simulink model "simulation"  (R2024b)
settings: Solver=FixedStepDiscrete  StartTime=0.0  StopTime=4  FixedStep=Ts  MaxStep=0.0001  RelTol=1e-3
PreLoadFcn:
  | load('parameters.m')
  | load('motor_parameters.m')
InitFcn:
  | if ~ evalin('base', 'exist(''A2'', ''var'')')
  |     load('all_parameters.mat');
  | end
values from neighbouring files (symbols this model uses):
  A1a = [0  0.0011361488425; -0.0011361488425  0]    [all_parameters.mat]    (also in parameters.m = [0 a12; a21 0])
  A1d = [0.987343830616  0; 0  0.987343830616]    [all_parameters.mat]    (also in parameters.m = [a11 0; 0 a22])
  A2 = [0.87358490566  0; 0  0.87358490566]    [all_parameters.mat]    (also in parameters.m = [a33, 0; 0, a44])
  A3a = [0  -0.00121090521585; 0.00121090521585  0]    [all_parameters.mat]    (also in parameters.m = [0 a52; a61 0])
  A3d = [-0.0123977153824  0; 0  -0.0123977153824]    [all_parameters.mat]    (also in parameters.m = [a51 0; 0 a62])
  B1 = [0.00755592202018  0; 0  0.00755592202018]    [all_parameters.mat]    (also in parameters.m = [b1, 0; 0, b1]*4)
  B1_inv = [132.346522017  0; 0  132.346522017]    [all_parameters.mat]    (also in parameters.m = inv(B1))
  B2 = [0.0188679245283  0; 0  0.0188679245283]    [all_parameters.mat]    (also in parameters.m = [b2, 0; 0, b2])
  B2_inv = [53  0; 0  53]    [all_parameters.mat]    (also in parameters.m = inv(B2))
  B3 = [-0.00740162112379  0; 0  -0.00740162112379]    [all_parameters.mat]    (also in parameters.m = [b3, 0; 0, b3]*4)
  Bm = 0.0024    [all_parameters.mat]    (also in parameters.m)
  gamma = [0.9  0; 0  0.9]    [all_parameters.mat]    (also in parameters.m = diag(v_gamma))
  H1a = [0  0.0011598340301; -0.0011598340301  0]    [all_parameters.mat]    (also in parameters.m = [0 h12; h21 0])
  H1d = [0.0127677964385  0; 0  0.0127677964385]    [all_parameters.mat]    (also in parameters.m = [h11 0; 0 h22])
  H2a = [0  -0.0012361488425; 0.0012361488425  0]    [all_parameters.mat]    (also in parameters.m = [0 h32; h41 0])
  H2d = [0.986392107509  0; 0  0.986392107509]    [all_parameters.mat]    (also in parameters.m = [h31 0; 0 h42])
  Jm_ = 2.38095238095    [all_parameters.mat]    (also in parameters.m)
  lambda = [0.5  0; 0  0.5]    [all_parameters.mat]    (also in parameters.m = diag(v_lambda))
  Lr = 0.6268    [all_parameters.mat]    (also in parameters.m)
  M_ind = 0.1535    [all_parameters.mat]    (also in parameters.m)
  P = 1    [all_parameters.mat]    (also in parameters.m)
  rho = [30  0; 0  30]    [all_parameters.mat]    (also in parameters.m = [rho1 0; 0 rho2])
  Rr = 6.9    [all_parameters.mat]    (also in parameters.m)
  T_inv = [1 0.866025403784 -0.5 -0.866025403784 -0.5 0 0 0.5 0.866025403784 0.5 -0.866025403784 -1 ... (36 elements, 6x6)]    [all_parameters.mat]    (also in parameters.m = inv(T))
  Tl = 2    [all_parameters.mat]    (also in parameters.m)
  Ts = 0.0001    [all_parameters.mat]    (also in parameters.m)
undefined symbols (not defined in the file or in its folder): rad, s
libraries: aerolibconvert2 x2, simulink x2, slpidlib x1, mcbcontrolslib x1
settings Model: Creator=bojack  LastModifiedBy=bojack

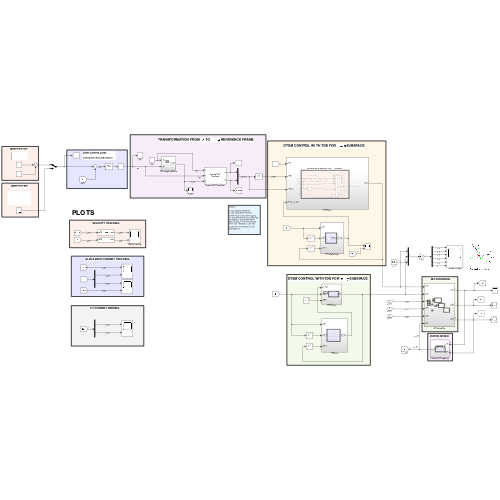
[thumbnail: Simulink's stored preview of the top-level diagram]
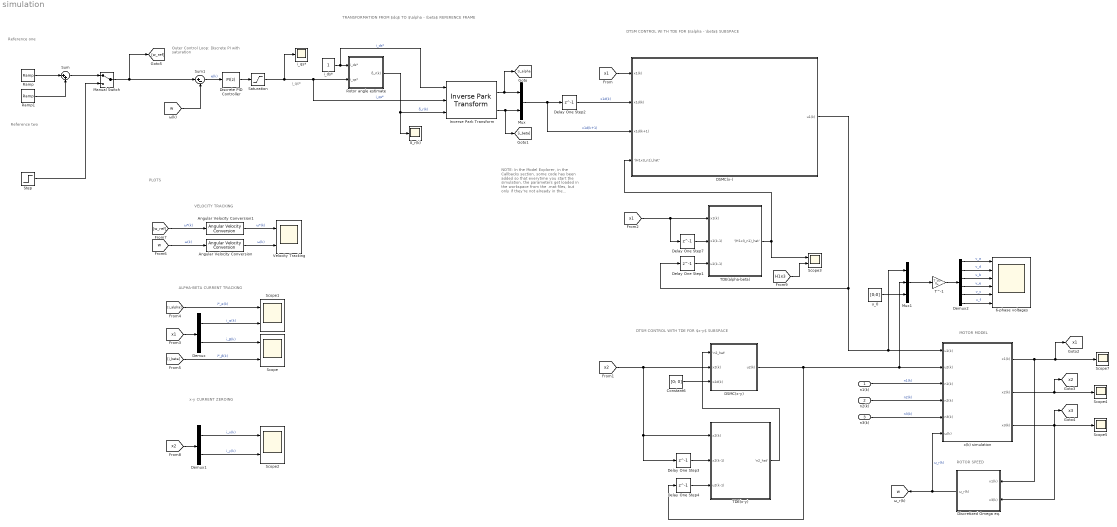
== system simulation ==
  note: Reference one
  note: VELOCITY TRACKING
  note: PLOTS
  note: Outer Control Loop:
      |
      | Discrete PI with saturation
  note: i_qs*
  note: NOTE:
      |
      | In the Model Explorer,
      | in the Callbacks section,
      | some code has been added
      | so that everytime you start the
      | simulation, the parameters
      | get loaded in the workspace
      | from the .mat files, but only
      | if they're not already in the
      | Workspace.
  note: DTSM CONTROL WITH TDE FOR $x-y$ SUBSPACE
  note: DTSM CONTROL WI TH TDE FOR $\alpha - \beta$ SUBSPACE
  note: TRANSFORMATION FROM $dq$ TO $\alpha - \beta$ REFERENCE FRAME
  note: ALPHA-BETA CURRENT TRACKING
  note: x-y CURRENT ZEROING
  note: MOTOR MODEL
  note: ROTOR SPEED
  note: Reference two
  n1(k) : Inport
  n2(k) : Inport  Port=2
  n3(k) : Inport  Port=3
  6-phase voltages : Scope  NumInputPorts=6
  Angular Velocity Conversion : aerolibconvert2/Angular Velocity Conversion  IU=rad/s  OU=rpm
  Angular Velocity Conversion1 : aerolibconvert2/Angular Velocity Conversion  IU=rad/s  OU=rpm
  Constant6 : Constant  Value=[0; 0]
  DSMC(x-) : Subsystem
  DSMC(x-y) : Subsystem
  Delay One Step1 : Delay  DelayLength=1  InitialCondition=[0 0]  SampleTime=Ts
  Delay One Step2 : Delay  DelayLength=1
  Delay One Step3 : Delay  DelayLength=1  InitialCondition=[0 0]
  Delay One Step4 : Delay  DelayLength=1  InitialCondition=[0 0]
  Delay One Step7 : Delay  DelayLength=1  InitialCondition=[0 0]
  Demux : Demux  Outputs=2
  Demux1 : Demux  Outputs=2
  Demux2 : Demux  Outputs=6
  Discrete PID Controller : slpidlib/PID Controller  Controller=PI  Form=Parallel  TimeDomain=Discrete-time  UseExternalTs=off  SampleTime=Ts  IntegratorMethod=Forward Euler  FilterMethod=Forward Euler  ControllerParametersSource=internal  P=0.9  I=0.027  UseKiTs=off  D=0  UseExternalDerivativeSource=off  N=100  UseFilter=on  TunerSelectOption=Transfer Function Based (PID Tuner App)  InitialConditionSource=internal  InitialConditionForIntegrator=0  InitialConditionForFilter=0  DifferentiatorICPrevScaledInput=0  ExternalReset=none  TrackingMode=off  Kt=1  LimitOutput=off  SatLimitsSource=internal  UpperSaturationLimit=inf  LowerSaturationLimit=-inf  LinearizeAsGain=off  AntiWindupMode=none  Kb=1  LimitIntegrator=off  UpperIntegratorSaturationLimit=inf  LowerIntegratorSaturationLimit=-inf  POutMin=[]  POutMax=[]  IOutMin=[]  IOutMax=[]  DOutMin=[]  DOutMax=[]  NOutMin=[]  NOutMax=[]  SumOutMin=[]  SumOutMax=[]  SaturationOutMin=[]  SaturationOutMax=[]  PParamMin=[]  PParamMax=[]  IParamMin=[]  IParamMax=[]  DParamMin=[]  DParamMax=[]  NParamMin=[]  NParamMax=[]  KbParamMin=[]  KbParamMax=[]  KtParamMin=[]  KtParamMax=[]  KbOutMin=[]  KbOutMax=[]  KtOutMin=[]  KtOutMax=[]  IntegratorOutMin=[]  IntegratorOutMax=[]  FilterOutMin=[]  FilterOutMax=[]  SumI1OutMin=[]  SumI1OutMax=[]  SumI2OutMin=[]  SumI2OutMax=[]  SumI3OutMin=[]  SumI3OutMax=[]  SumI4OutMin=[]  SumI4OutMax=[]  SumDOutMin=[]  SumDOutMax=[]  DifferentiatorOutMin=[]  DifferentiatorOutMax=[]  FilterDiffOutCoefMin=[]  FilterDiffOutCoefMax=[]  ReciprocalOutMin=[]  ReciprocalOutMax=[]  SumDenOutMin=[]  SumDenOutMax=[]  SumNumOutMin=[]  SumNumOutMax=[]  DivideOutMin=[]  DivideOutMax=[]  UdiffTsProdOutMin=[]  UdiffTsProdOutMax=[]  NTsProdOutMin=[]  NTsProdOutMax=[]  UintegralTsProdOutMin=[]  UintegralTsProdOutMax=[]  UngainTsProdOutMin=[]  UngainTsProdOutMax=[]  ClampingZeroOutDataTypeStr=Inherit: Inherit via back propagation  ClampingZeroOutMin=[]  ClampingZeroOutMax=[]  FilterDenConstantOutDataTypeStr=Inherit: Inherit via back propagation  FilterDenConstantOutMin=[]  FilterDenConstantOutMax=[]  PCopyOutDataTypeStr=Inherit: Inherit via back propagation  PCopyOutMin=[]  PCopyOutMax=[]  NCopyOutDataTypeStr=Inherit: Inherit via back propagation  NCopyOutMin=[]  NCopyOutMax=[]  IntegratorContinuousStateAttributes=''  IntegratorStateMustResolveToSignalObject=off  IntegratorRTWStateStorageClass=Auto  FilterContinuousStateAttributes=''  FilterStateMustResolveToSignalObject=off  FilterRTWStateStorageClass=Auto  ParallelPVariant=InternalParameters  IdealPVariant=Disabled  IVariant=InternalParameters  DVariant=Disabled  IntegratorVariant=Discrete  SatVariant=Disabled  AWVariant=Passthrough  PCopyVariant=Disabled  TRVariant=Disabled  FdbkBlocksVariant=Forward  IdealPFdbkVariant=Disabled  SatFdbkVariant=Disabled  DerivativeFilterVariant=Disabled  NVariant=Disabled  NCopyVariant=Disabled_SignalSpec  FilterICVariant=Disabled  IntegratorICVariant=InternalICs  ExternalResetVariant=Disabled  TRSumVariant=Passthrough  SumFdbkVariant=Disabled  SumVariant=Sum_PI  TsampFilterVariant=InternalTs  TsampNgainVariant=Passthrough  TsampIntegralVariant=Disabled_SignalSpec  ExternalSaturationOutDataTypeStr=Inherit: Same as second input  DerivativeSourceVariant=Disabled  PreIntVariant=InternalPreInt
      settings: LibrarySourceBlock=simulink/Discrete/Discrete PID Controller
  Discretized Omega eq. : Subsystem
  Inverse Park Transform : mcbcontrolslib/Inverse Park Transform  PhaseInput=Two inputs  AxisAlignment=D-axis  ThetaInput=Electrical position  AngleInput=Radians  N_points=1024
      settings: LibrarySourceBlock=mcbhdllib/Controls/Math Transforms/Inverse Park Transform
  Manual Switch : ManualSwitch
  Mux : Mux  Inputs=2
  Mux1 : Mux  Inputs=3
  Ramp : simulink/Sources/Ramp  slope=157/2  start=0  InitialOutput=0
  Ramp1 : simulink/Sources/Ramp  slope=-157/2  start=2  InitialOutput=0
  Rotor angle estimate : Subsystem
  Saturation : Saturate  UpperLimit=5  LowerLimit=-5
  Scope{,1..3} (4 alike) : Scope  NumInputPorts=2
  Scope4 : Scope
  Scope5 : Scope
  Scope7 : Scope
  Step : Step  Time=2  Before=52  After=-52  SampleTime=Ts
  Sum : Sum  Inputs=|++
  Sum1 : Sum  Inputs=|+-
  TDE(alpha-beta) : Subsystem
  TDE(x-y) : Subsystem
  T^-1 : Gain  Gain=T_inv  Multiplication=Matrix(K*u)
  Velocity Tracking : Scope  NumInputPorts=2
  i_ds* : Constant
  i_qs* : Scope
  u_0 : Constant  Value=[0;0]
  x(k) simulation : Subsystem
  δ_r(k) : Scope
  tag scope: w=global, x1=global, x2=global, x3=global
  wires:
  n2(k)/1 -> x(k) simulation/4(n2(k))  "n2(k)"
  n1(k)/1 -> x(k) simulation/3(n1(k))  "n1(k)"
  Discretized Omega eq./1(ω_r(k)) -> x(k) simulation/6(ω(k)), [w]  "ω_r(k)"
  n3(k)/1 -> x(k) simulation/5(n3(k))  "n3(k)"
  x(k) simulation/2(x2(k)) -> Scope4/1, [x2]
  DSMC(x-y)/1(u2(k)) -> Delay One Step4/1, Mux1/2, x(k) simulation/2(u2(k))
  x(k) simulation/1(x1(k)) -> Discretized Omega eq./1(x1(k)), Scope7/1, [x1]
  DSMC(x-)/1(u1(k)) -> Mux1/1, x(k) simulation/1(u1(k)), Delay One Step1/1
  TDE(alpha-beta)/1("'(H1x3_n1)_hat' ") -> Scope3/1, DSMC(x-)/4("'(H1x3_n1)_hat' ")
  Delay One Step7/1 -> TDE(alpha-beta)/2(x1(k-1))
  Delay One Step1/1 -> TDE(alpha-beta)/3(u1(k-1))
  Sum1/1 -> Discrete PID Controller/1  "e(k)"
  Inverse Park Transform/1 -> [i_alpha], Mux/1
  i_ds*/1 -> Inverse Park Transform/1, Rotor angle estimate/1(i_ds*)  "i_ds*"
  Discrete PID Controller/1 -> Saturation/1
  Inverse Park Transform/2 -> [i_beta], Mux/2
  [w] -> Sum1/2
  Rotor angle estimate/1(δ_r(k)) -> Inverse Park Transform/3, δ_r(k)/1  "δ_r(k)"
  Mux/1 -> DSMC(x-)/3(x1d(k+1)), Delay One Step2/1  "x1d(k+1)"
  Delay One Step2/1 -> DSMC(x-)/2(x1d(k))  "x1d(k)"
  Saturation/1 -> Inverse Park Transform/2, Rotor angle estimate/2(i_qs*), i_qs*/1  "i_qs*"
  x(k) simulation/3(x3(k)) -> Discretized Omega eq./2(x3(k)), Scope5/1, [x3]
  [x1] -> DSMC(x-)/1(x1(k))
  [x1] -> TDE(alpha-beta)/1(x1(k)), Delay One Step7/1
  [x2] -> Delay One Step3/1, TDE(x-y)/1(x2(k)), DSMC(x-y)/2(x2(k))
  Delay One Step4/1 -> TDE(x-y)/3(u2(k-1))
  Constant6/1 -> DSMC(x-y)/3(x2d(k))
  Delay One Step3/1 -> TDE(x-y)/2(x2(k-1))
  TDE(x-y)/1("'n2_hat' ") -> DSMC(x-y)/1("'n2_hat' ")
  [x1] -> Demux/1
  Demux/2 -> Scope/1  "i_β(k)"
  [i_beta] -> Scope/2  "i*_β(k)"
  Demux/1 -> Scope1/2  "i_α(k)"
  [i_alpha] -> Scope1/1  "i*_α(k)"
  [w_ref] -> Angular Velocity Conversion1/1  "ω*(k)"
  [w] -> Angular Velocity Conversion/1  "ω(k)"
  Angular Velocity Conversion1/1 -> Velocity Tracking/1  "ω*(k)"
  Angular Velocity Conversion/1 -> Velocity Tracking/2  "ω(k)"
  Demux1/2 -> Scope2/2  "i_y(k)"
  Demux1/1 -> Scope2/1  "i_x(k)"
  [x2] -> Demux1/1
  u_0/1 -> Mux1/3
  Mux1/1 -> T^-1/1
  T^-1/1 -> Demux2/1
  Demux2/4 -> 6-phase voltages/4  "v_e"
  Demux2/3 -> 6-phase voltages/3  "v_b"
  Demux2/2 -> 6-phase voltages/2  "v_d"
  Demux2/1 -> 6-phase voltages/1  "v_a"
  Demux2/5 -> 6-phase voltages/5  "v_c"
  Demux2/6 -> 6-phase voltages/6  "v_f"
  Ramp/1 -> Sum/1
  Ramp1/1 -> Sum/2
  [H1x3] -> Scope3/2
  Step/1 -> Manual Switch/2
  Sum/1 -> Manual Switch/1
  Manual Switch/1 -> Sum1/1, [w_ref]

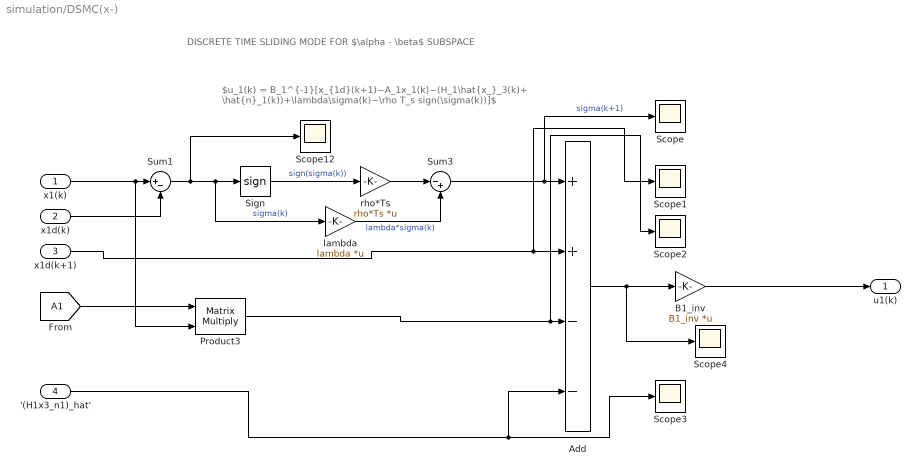
== system simulation/DSMC(x-) ==
  note: DISCRETE TIME SLIDING MODE FOR $\alpha - \beta$ SUBSPACE
  note: $u_1(k) = B_1^{-1}[x_{1d}(k+1)−A_1x_1(k)−(H_1\hat{x_}_3(k)+ \hat{n}_1(k))+\lambda\sigma(k)−\rho T_s sign(\sigma(k))]$
  x1(k) : Inport
  x1d(k) : Inport  Port=2
  x1d(k+1) : Inport  Port=3  PortDimensions=2
  "'(H1x3_n1)_hat' " : Inport  Port=4
  Add : Sum  Inputs=++--
  B1_inv : Gain  Gain=B1_inv  Multiplication=Matrix(K*u)
  Product3 : Product  Multiplication=Matrix(*)
  Scope{,1..4,12} (6 alike) : Scope
  Sign : Signum
  Sum1 : Sum  Inputs=|+-
  Sum3 : Sum  Inputs=|-+
  lambda : Gain  Gain=lambda  Multiplication=Matrix(K*u)
  rho*Ts : Gain  Gain=rho*Ts  Multiplication=Matrix(K*u)
  u1(k) : Outport
  wires:
  Product3/1 -> Scope2/1, Add/3
  x1d(k)/1 -> Sum1/2
  Sum3/1 -> Scope/1, Add/1  "sigma(k+1)"
  x1(k)/1 -> Product3/2, Sum1/1
  Sum1/1 -> Scope12/1, lambda/1, Sign/1  "sigma(k)"
  Sign/1 -> rho*Ts/1  "sign(sigma(k))"
  [A1] -> Product3/1
  rho*Ts/1 -> Sum3/1
  Add/1 -> Scope4/1, B1_inv/1
  lambda/1 -> Sum3/2  "lambda*sigma(k)"
  x1d(k+1)/1 -> Scope1/1, Add/2
  "'(H1x3_n1)_hat' "/1 -> Scope3/1, Add/4
  B1_inv/1 -> u1(k)/1

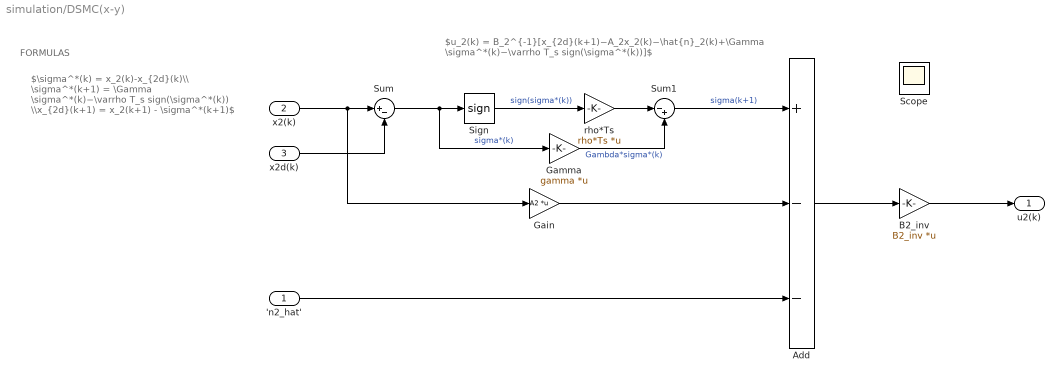
== system simulation/DSMC(x-y) ==
  note: $u_2(k) = B_2^{-1}[x_{2d}(k+1)−A_2x_2(k)−\hat{n}_2(k)+\Gamma \sigma^*(k)−\varrho T_s sign(\sigma^*(k))]$
  note: $\sigma^*(k) = x_2(k)-x_{2d}(k)\\ \sigma^*(k+1) = \Gamma \sigma^*(k)−\varrho T_s sign(\sigma^*(k)) \\x_{2d}(k+1) = x_2(k+1) - \sigma^*(k+1)$
  note: FORMULAS
  "'n2_hat' " : Inport
  x2(k) : Inport  Port=2
  x2d(k) : Inport  Port=3
  Add : Sum  Inputs=+--
  B2_inv : Gain  Gain=B2_inv  Multiplication=Matrix(K*u)
  Gain : Gain  Gain=A2  Multiplication=Matrix(K*u)
  Gamma : Gain  Gain=gamma  Multiplication=Matrix(K*u)
  Scope : Scope
  Sign : Signum
  Sum : Sum  Inputs=|+-
  Sum1 : Sum  Inputs=|-+
  rho*Ts : Gain  Gain=rho*Ts  Multiplication=Matrix(K*u)
  u2(k) : Outport
  wires:
  Gain/1 -> Add/2
  B2_inv/1 -> u2(k)/1
  Add/1 -> B2_inv/1
  x2(k)/1 -> Gain/1, Sum/1
  Sum/1 -> Gamma/1, Sign/1  "sigma*(k)"
  "'n2_hat' "/1 -> Add/3
  Sign/1 -> rho*Ts/1  "sign(sigma*(k))"
  x2d(k)/1 -> Sum/2
  Sum1/1 -> Add/1  "sigma(k+1)"
  rho*Ts/1 -> Sum1/1
  Gamma/1 -> Sum1/2  "Gambda*sigma*(k)"

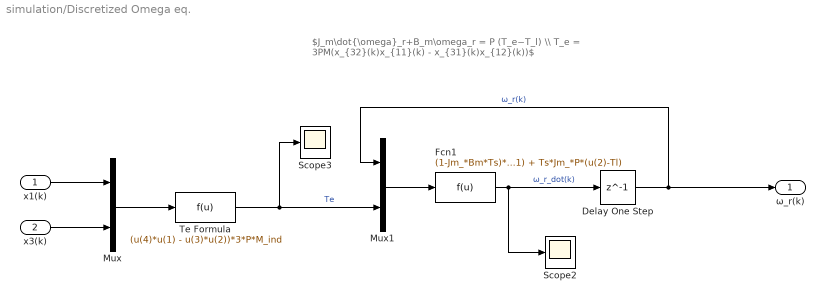
== system simulation/Discretized Omega eq. ==
  note: $J_m\dot{\omega}_r+B_m\omega_r = P (T_e−T_l) \\ T_e = 3PM(x_{32}(k)x_{11}(k) - x_{31}(k)x_{12}(k))$
  x1(k) : Inport  PortDimensions=2
  x3(k) : Inport  Port=2  PortDimensions=2
  Delay One Step : Delay  DelayLength=1
  Fcn1 : Fcn  Expr=(1-Jm_*Bm*Ts)*u(1) + Ts*Jm_*P*(u(2)-Tl)
  Mux : Mux  Inputs=2
  Mux1 : Mux  Inputs=2
  Scope2 : Scope
  Scope3 : Scope
  Te Formula : Fcn  Expr=(u(4)*u(1) - u(3)*u(2))*3*P*M_ind
  ω_r(k) : Outport  PortDimensions=1
  wires:
  Fcn1/1 -> Scope2/1, Delay One Step/1  "ω_r_dot(k)"
  Delay One Step/1 -> ω_r(k)/1, Mux1/1  "ω_r(k)"
  Te Formula/1 -> Scope3/1, Mux1/2  "Te"
  x1(k)/1 -> Mux/1
  x3(k)/1 -> Mux/2
  Mux/1 -> Te Formula/1
  Mux1/1 -> Fcn1/1

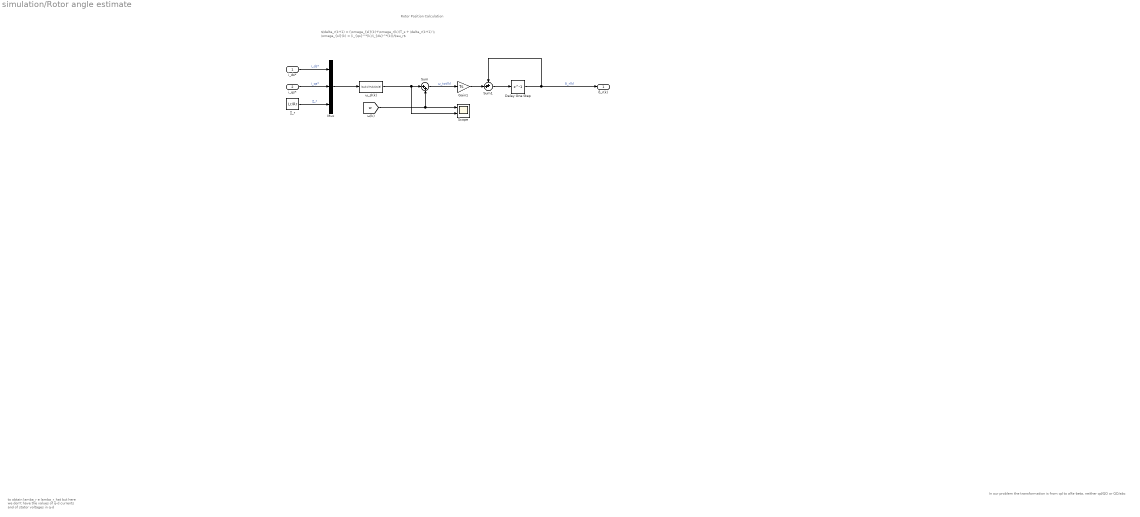
== system simulation/Rotor angle estimate ==
  note: $\delta_r(k+1) = (\omega_{sl}(k)+\omega_r(k))T_s + \delta_r(k+1) \\ \omega_{sl}(k) = (i_{qs}^*(k)/i_{ds}^*(k))/\tau_r$
  note: Rotor Position Calculation
  note: In our problem the transformation is from qd to alfa-beta, neither qd/QD or QD/abc
  note: to obtain lamba_r e lamba_r_hat
      | but here we don't have the values of
      | q-d currents and of stator voltages in q-d
  i_ds* : Inport
  i_qs* : Inport  Port=2
  Delay One Step : Delay  DelayLength=1
  Gain1 : Gain  Gain=Ts
  Mux : Mux  Inputs=3
  Scope : Scope  NumInputPorts=2
  Sum : Sum  Inputs=|++
  Sum1 : Sum  Inputs=++|
  ω_sl(k) : Fcn  Expr=(1/u(1))*u(2)/u(3)
  𝜏_r : Constant  Value=Lr/Rr
  δ_r(k) : Outport
  wires:
  [w] -> Sum/2, Scope/1
  Sum/1 -> Gain1/1  "ω_tot(k)"
  i_ds*/1 -> Mux/1  "i_ds*"
  i_qs*/1 -> Mux/2  "i_qs*"
  Mux/1 -> ω_sl(k)/1
  ω_sl(k)/1 -> Sum/1, Scope/2
  𝜏_r/1 -> Mux/3  "𝜏_r"
  Gain1/1 -> Sum1/2
  Delay One Step/1 -> Sum1/1, δ_r(k)/1  "δ_r(k)"
  Sum1/1 -> Delay One Step/1

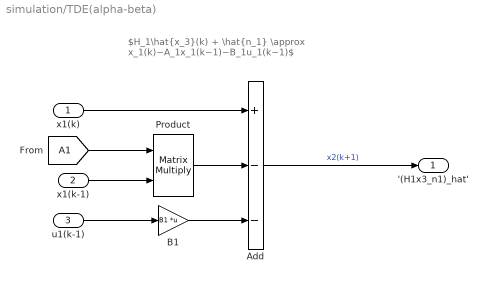
== system simulation/TDE(alpha-beta) ==
  note: $H_1\hat{x_3}(k) + \hat{n_1} \approx x_1(k)−A_1x_1(k−1)−B_1u_1(k−1)$
  x1(k) : Inport
  x1(k-1) : Inport  Port=2  PortDimensions=2
  u1(k-1) : Inport  Port=3  PortDimensions=2
  Add : Sum  Inputs=+--
  B1 : Gain  Gain=B1  Multiplication=Matrix(K*u)
  Product : Product  Multiplication=Matrix(*)
  "'(H1x3_n1)_hat' " : Outport
  wires:
  x1(k-1)/1 -> Product/2
  u1(k-1)/1 -> B1/1
  x1(k)/1 -> Add/1
  Product/1 -> Add/2
  B1/1 -> Add/3
  Add/1 -> "'(H1x3_n1)_hat' "/1  "x2(k+1)"
  [A1] -> Product/1

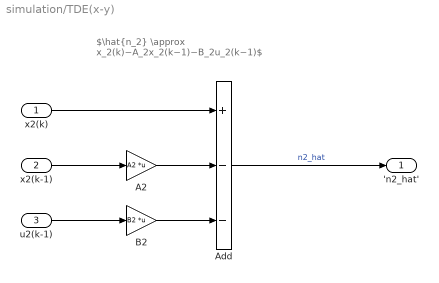
== system simulation/TDE(x-y) ==
  note: $\hat{n_2} \approx x_2(k)−A_2x_2(k−1)−B_2u_2(k−1)$
  x2(k) : Inport
  x2(k-1) : Inport  Port=2
  u2(k-1) : Inport  Port=3
  A2 : Gain  Gain=A2  Multiplication=Matrix(K*u)
  Add : Sum  Inputs=+--
  B2 : Gain  Gain=B2  Multiplication=Matrix(K*u)
  "'n2_hat' " : Outport
  wires:
  B2/1 -> Add/3
  Add/1 -> "'n2_hat' "/1  "n2_hat"
  x2(k)/1 -> Add/1
  u2(k-1)/1 -> B2/1
  A2/1 -> Add/2
  x2(k-1)/1 -> A2/1

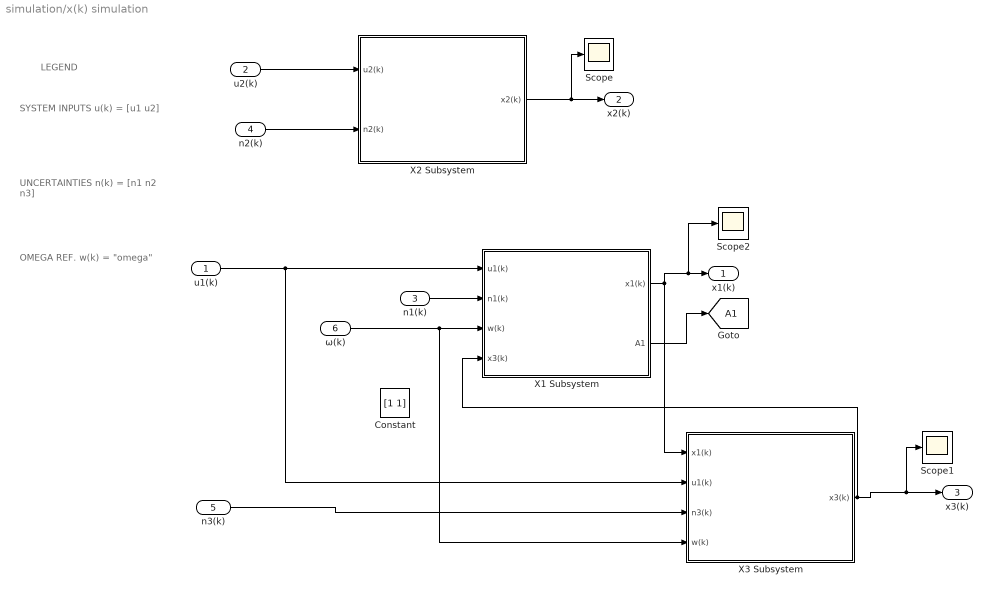
== system simulation/x(k) simulation ==
  note: LEGEND
  note: SYSTEM INPUTS
      |
      | u(k) = [u1 u2]
  note: UNCERTAINTIES
      |
      | n(k) = [n1 n2 n3]
  note: OMEGA REF.
      |
      | w(k) = "omega"
  u1(k) : Inport
  u2(k) : Inport  Port=2
  n1(k) : Inport  Port=3  PortDimensions=2
  n2(k) : Inport  Port=4  PortDimensions=2
  n3(k) : Inport  Port=5  PortDimensions=2
  ω(k) : Inport  Port=6
  Constant : Constant  Value=[1 1]
  Scope : Scope
  Scope1 : Scope
  Scope2 : Scope
  X1 Subsystem : Subsystem
  X2 Subsystem : Subsystem
  X3 Subsystem : Subsystem
  x1(k) : Outport
  x2(k) : Outport  Port=2
  x3(k) : Outport  Port=3
  tag scope: A1=global
  wires:
  n1(k)/1 -> X1 Subsystem/2(n1(k))
  n3(k)/1 -> X3 Subsystem/3(n3(k))
  X2 Subsystem/1(x2(k)) -> Scope/1, x2(k)/1
  ω(k)/1 -> X3 Subsystem/4(w(k)), X1 Subsystem/3(w(k))
  u1(k)/1 -> X3 Subsystem/2(u1(k)), X1 Subsystem/1(u1(k))
  X1 Subsystem/1(x1(k)) -> Scope2/1, x1(k)/1, X3 Subsystem/1(x1(k))
  X1 Subsystem/2(A1) -> [A1]
  u2(k)/1 -> X2 Subsystem/1(u2(k))
  n2(k)/1 -> X2 Subsystem/2(n2(k))
  X3 Subsystem/1(x3(k)) -> X1 Subsystem/4(x3(k)), Scope1/1, x3(k)/1

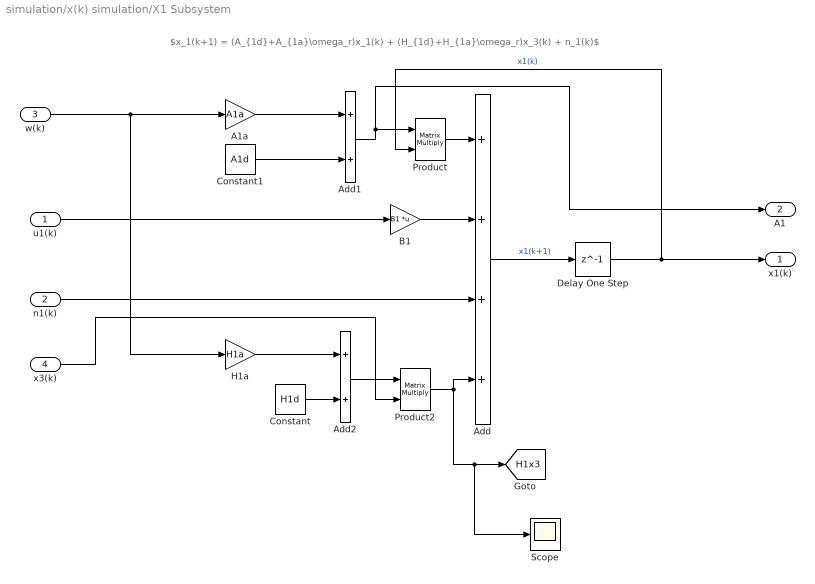
== system simulation/x(k) simulation/X1 Subsystem ==
  note: $x_1(k+1) = (A_{1d}+A_{1a}\omega_r)x_1(k) + (H_{1d}+H_{1a}\omega_r)x_3(k) + n_1(k)$
  u1(k) : Inport
  n1(k) : Inport  Port=2
  w(k) : Inport  Port=3
  x3(k) : Inport  Port=4  PortDimensions=2
  A1a : Gain  Gain=A1a
  Add : Sum  Inputs=++++
  Add1 : Sum
  Add2 : Sum
  B1 : Gain  Gain=B1  Multiplication=Matrix(K*u)
  Constant : Constant  Value=H1d
  Constant1 : Constant  Value=A1d
  Delay One Step : Delay  DelayLength=1  InitialCondition=[0 0]
  H1a : Gain  Gain=H1a
  Product : Product  Multiplication=Matrix(*)
  Product2 : Product  Multiplication=Matrix(*)
  Scope : Scope
  x1(k) : Outport
  A1 : Outport  Port=2  PortDimensions=[2,2]
  tag scope: H1x3=global
  wires:
  u1(k)/1 -> B1/1
  B1/1 -> Add/2
  Add/1 -> Delay One Step/1  "x1(k+1)"
  Delay One Step/1 -> Product/2, x1(k)/1  "x1(k)"
  n1(k)/1 -> Add/3
  Constant1/1 -> Add1/2
  w(k)/1 -> H1a/1, A1a/1
  Add1/1 -> Product/1, A1/1
  H1a/1 -> Add2/1
  Constant/1 -> Add2/2
  A1a/1 -> Add1/1
  Product2/1 -> Scope/1, [H1x3], Add/4
  Add2/1 -> Product2/1
  x3(k)/1 -> Product2/2
  Product/1 -> Add/1

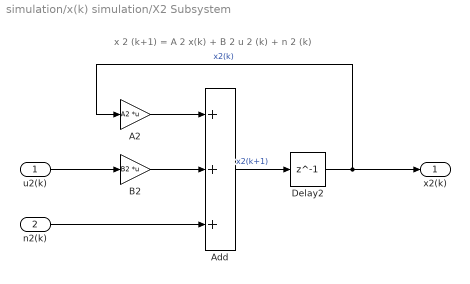
== system simulation/x(k) simulation/X2 Subsystem ==
  note: x 2 (k+1) = A 2 x(k) + B 2 u 2 (k) + n 2 (k)
  u2(k) : Inport
  n2(k) : Inport  Port=2
  A2 : Gain  Gain=A2  Multiplication=Matrix(K*u)
  Add : Sum  Inputs=+++
  B2 : Gain  Gain=B2  Multiplication=Matrix(K*u)
  Delay2 : Delay  DelayLength=1  InitialCondition=[0; 0]
  x2(k) : Outport
  wires:
  u2(k)/1 -> B2/1
  B2/1 -> Add/2
  A2/1 -> Add/1
  n2(k)/1 -> Add/3
  Add/1 -> Delay2/1  "x2(k+1)"
  Delay2/1 -> x2(k)/1, A2/1  "x2(k)"

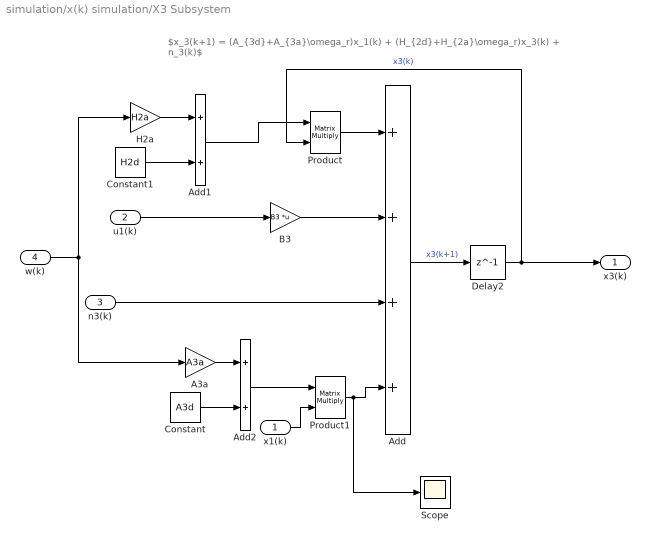
== system simulation/x(k) simulation/X3 Subsystem ==
  note: $x_3(k+1) = (A_{3d}+A_{3a}\omega_r)x_1(k) + (H_{2d}+H_{2a}\omega_r)x_3(k) + n_3(k)$
  x1(k) : Inport
  u1(k) : Inport  Port=2
  n3(k) : Inport  Port=3
  w(k) : Inport  Port=4
  A3a : Gain  Gain=A3a
  Add : Sum  Inputs=++++
  Add1 : Sum
  Add2 : Sum
  B3 : Gain  Gain=B3  Multiplication=Matrix(K*u)
  Constant : Constant  Value=A3d
  Constant1 : Constant  Value=H2d
  Delay2 : Delay  DelayLength=1  InitialCondition=[0 0]
  H2a : Gain  Gain=H2a
  Product : Product  Multiplication=Matrix(*)
  Product1 : Product  Multiplication=Matrix(*)
  Scope : Scope
  x3(k) : Outport
  wires:
  u1(k)/1 -> B3/1
  B3/1 -> Add/2
  Add/1 -> Delay2/1  "x3(k+1)"
  Delay2/1 -> Product/2, x3(k)/1  "x3(k)"
  n3(k)/1 -> Add/3
  w(k)/1 -> H2a/1, A3a/1
  Constant/1 -> Add2/2
  H2a/1 -> Add1/1
  Constant1/1 -> Add1/2
  Product/1 -> Add/1
  Product1/1 -> Scope/1, Add/4
  Add2/1 -> Product1/1
  x1(k)/1 -> Product1/2
  A3a/1 -> Add2/1
  Add1/1 -> Product/1
